simulink model "lqg_cartpend_sim_modified"  (R2015a)
settings: Solver=ode45  StartTime=0.0  StopTime=50.0  RelTol=1e-3
values from neighbouring files (symbols this model uses):
  C = cos( y(:,3) )    [cartPendMatrix.m]    (also in cartPendVector.m = cos( y(3) ); run_cartPend_LQG.m = [1 1 1 1]; run_cartPend_kalmanFilter.m = [1 0 0 0]; run_cartPend_obs.m = [0 1 0 0])
  K = place(A, B, p )    [run_cartPend.m]    (also in run_cartPend_LQG.m = [0,0,0,0]; run_cartPend_LQR.m = lqr( A,B,Q,R); run_cartPend_linearizedControl.m; simulink_cartPend_initialize.m = [0,0,0,0])
  sysKF = ss(A-Lmat*C,[B Lmat],eye(4),0*[B Lmat])    [run_cartPend_LQG.m]    (also in run_cartPend_kalmanFilter.m = ss(A-Kf*C,[B Kf],eye(4),0*[B Kf]))
settings Model: Creator=sbrunton  LastModifiedBy=Thomas
settings DataIOCC: SaveFormat=Dataset
settings HardwareCC: ProdBitPerPointer=64  ProdLargestAtomicFloat=Float  ProdIntDivRoundTo=Zero  ProdEndianess=LittleEndian  ProdWordSize=64  ProdHWDeviceType=Intel->x86-64 (Windows64)
settings GRTTargetCC: GeneratePreprocessorConditionals=Use local settings
settings ConfigComp: CovMetricSettings=dw  CovHtmlReporting=on  CovSaveCumulativeToWorkspaceVar=on  CovSaveSingleToWorkspaceVar=on  CovExternalEMLEnable=off

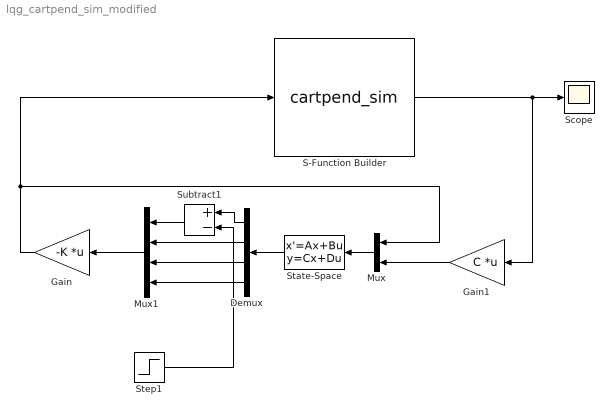
== system lqg_cartpend_sim_modified ==
  Demux : Demux
  Gain : Gain  Gain=-K  Multiplication=Matrix(K*u) (u vector)
  Gain1 : Gain  Gain=C  Multiplication=Matrix(K*u) (u vector)
  Mux : Mux  Inputs=2
  Mux1 : Mux
  S-Function Builder : S-Function  InitFcn=try, set_param(gcb,'FunctionName','cartpend_sim'), end  FunctionName=cartpend_sim  SFunctionModules=cartpend_sim_wrapper  mask(S-Function Builder){}
      mask help: Simulink:masks:SFunctionBuilder_MD
      mask init:
      | val = [[.9  0.75 0.75 1 1 .9 .9 1]',[1 1 0.75 0.75 .9 .9 1 .9]'];try , sys = get_param(gcb,'SfunBuilderFcnName');if isempty(sys), sys = get_param(gcb,'FunctionName'); end,catch, sys = get_param(gcb,'FunctionName'); end
      settings: CopyFcn=set_param(gcbh,'LinkStatus','none')  PreSaveFcn=try, set_param(gcb,'FunctionName','cartpend_sim'), end  OpenFcn=sfunctionwizard(gcbh)
      mask Display: plot(val(:,1),val(:,2)),disp(sys), port_label('input',1,'u0'), port_label('output',1,'y0')
  Scope : Scope
      settings: YMin=-0.59265  YMax=3.57093
  State-Space : StateSpace  A=sysKF.a  B=sysKF.b  C=sysKF.c  D=sysKF.d  X0=[0 0 0 0]
  Step1 : Step  Time=10  SampleTime=0
  Subtract1 : Sum  Inputs=+-
  wires:
  Gain/1 -> Mux/1, S-Function Builder/1
  S-Function Builder/1 -> Gain1/1, Scope/1
  Mux/1 -> State-Space/1
  Demux/2 -> Mux1/2
  Demux/4 -> Mux1/4
  Demux/3 -> Mux1/3
  Mux1/1 -> Gain/1
  Subtract1/1 -> Mux1/1
  Demux/1 -> Subtract1/1
  Step1/1 -> Subtract1/2
  State-Space/1 -> Demux/1
  Gain1/1 -> Mux/2
